simulink model "PI_Retour_Etat_LQR"  (R2024a)
settings: Solver=VariableStepAuto  StartTime=0.0  StopTime=10  RelTol=1e-3
undefined symbols (not defined in the file): A, B, K_lqr, x0
settings Model: Creator=DELL  LastModifiedBy=DELL

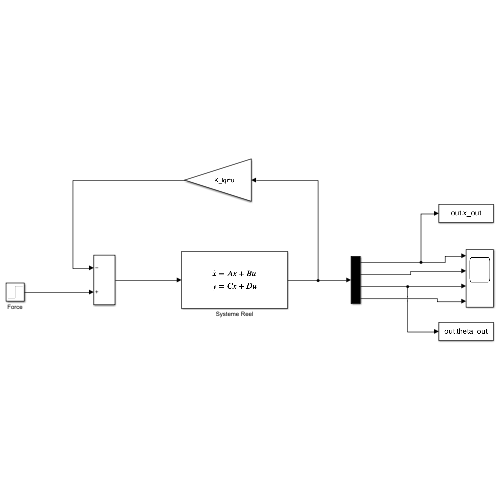
[thumbnail: Simulink's stored preview of the top-level diagram]
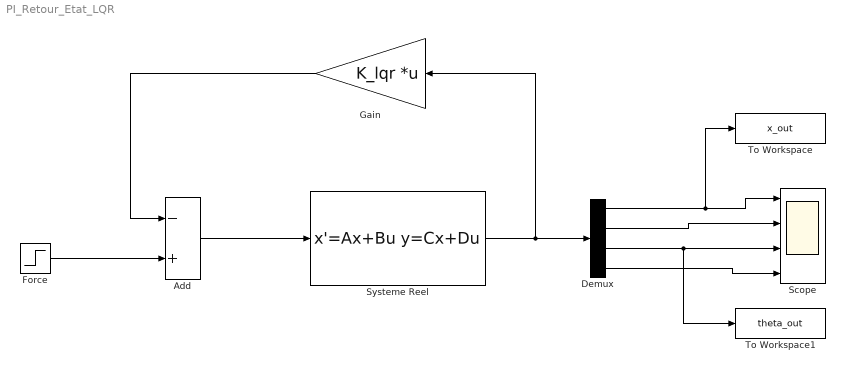
== system PI_Retour_Etat_LQR ==
  Add : Sum  Inputs=-+
  Demux : Demux
  Force : Step  Time=5  After=5  SampleTime=0
  Gain : Gain  Gain=K_lqr  Multiplication=Matrix(K*u)
  Scope : Scope  NumInputPorts=4
  Systeme Reel : StateSpace  A=A  B=B  C=eye(4);  D=zeros(4,1);  InitialCondition=x0
  To Workspace : ToWorkspace  VariableName=x_out  SaveFormat=Timeseries  SampleTime=-1
  To Workspace1 : ToWorkspace  VariableName=theta_out  SaveFormat=Timeseries  SampleTime=-1
  wires:
  Demux/1 -> To Workspace/1, Scope/1
  Gain/1 -> Add/1
  Force/1 -> Add/2
  Systeme Reel/1 -> Demux/1, Gain/1
  Demux/2 -> Scope/2
  Demux/3 -> To Workspace1/1, Scope/3
  Demux/4 -> Scope/4
  Add/1 -> Systeme Reel/1
